simulink model "Neurofeedback_Fuzzy_MISO_Full_3x3"  (R2022a)
settings: Solver=VariableStepAuto  StartTime=0.0  StopTime=2700  RelTol=1e-3
libraries: dspsrcs4 x12, simulink x5, fuzblock x1
(part 2 of 2)

== matlab function Neurofeedback_Fuzzy_MISO_Full_3x3/Synthetic Human Agent/Noise Models/Physiological Noise_ Vasomotion ==
  settings: updateMethod=DISCRETE
  data: FreqSD input; HemoNoises output; FreqMean input; ResolutionStep input; timestamps input
function HemoNoises  = Neurofeedback_PhysiologicalNoise(FreqSD, FreqMean, ResolutionStep, timestamps)
%% Version V1
% Authors - Mario De Los Santos, Felipe Orihuela-Espina, Javier
% Herrera-Vega, Javier Andreu-Pérez
% Date - July 18th, 2022
% Email - madlsh3517@gmail.com
% Based on: Elwell et. al., 1999. Oscillations in cerebal haemodynamics.
%
%% Input Parameters
% FreqSD - Frequency standard deviation of the physiological noise. Scalar
% FreqMean - Frequency Mean of the physiological noise. Scalar
% Resolution Step - Sampling rate. Scalar
% Timestamps - Time sequence for the stimulus train. <1 x simulationLength>
% NRegions - Number of regions activated. Scalar.
%% Output Parameters
% 
% HemoNoises -  Noise generation for the hemodynamics signals.
%               <NRegions x simulationLength>
%
%% 

%Variables to ADD the noises to the models. 
% These variables divide the hemodynamics 
% inputs depending on the number of regions.
HemoNoises = 0;

%Calculation of the operative ranges to use
Initial =  FreqMean - 2 * FreqSD;
Ending = FreqMean + 2 * FreqSD + ResolutionStep;
Calsize =  (Ending - Initial)/ResolutionStep;
FrequencySet = linspace(Initial, Ending, Calsize);

amplitudeScaling = 1;
for i = 1:Calsize
    s = rng; %Rebot random seeed 
    %Random Amplitude
    %Centralized gaussian in the dispersion mean 
    %A = 0;
    A = amplitudeScaling * normrnd(FreqMean,FreqSD);
    %A = amplitudeScaling * randn(1);
  
    %Random phase
    theta = (2 * pi * normrnd(FreqMean, FreqSD) - pi );
  
    %Fundamental signal
    tmpSin = A * sin(pi * FrequencySet(1,i) * timestamps + theta);
    HemoNoises = HemoNoises + tmpSin;
end
%This section should be generalized but do the work for now.

== matlab function Neurofeedback_Fuzzy_MISO_Full_3x3/Synthetic Human Agent/Noise Models/Physiological Noise_Heart ==
  settings: updateMethod=DISCRETE
  data: FreqSD input; HemoNoises output; FreqMean input; ResolutionStep input; timestamps input
function HemoNoises  = Neurofeedback_PhysiologicalNoise(FreqSD, FreqMean, ResolutionStep, timestamps)
%% Version V1
% Authors - Mario De Los Santos, Felipe Orihuela-Espina, Javier
% Herrera-Vega, Javier Andreu-Pérez
% Date - July 18th, 2022
% Email - madlsh3517@gmail.com
% Based on: Elwell et. al., 1999. Oscillations in cerebal haemodynamics.
%
%% Input Parameters
% FreqSD - Frequency standard deviation of the physiological noise. Scalar
% FreqMean - Frequency Mean of the physiological noise. Scalar
% Resolution Step - Sampling rate. Scalar
% Timestamps - Time sequence for the stimulus train. <1 x simulationLength>
% NRegions - Number of regions activated. Scalar.
%% Output Parameters
% 
% HemoNoises -  Noise generation for the hemodynamics signals.
%               <NRegions x simulationLength>
%
%% 

%Variables to ADD the noises to the models. 
% These variables divide the hemodynamics 
% inputs depending on the number of regions.
HemoNoises = 0;
%
%Calculation of the operative ranges to use
Initial =  FreqMean - 2*FreqSD;
Ending = FreqMean +  2*FreqSD;
Calsize = (Ending - Initial - ResolutionStep)/ResolutionStep;
%Calsize = ResolutionStep;
FrequencySet = linspace(Initial, Ending, Calsize);

amplitudeScaling = 1;
theta = 0;
for i = 1:Calsize
    s = rng; %Rebot random seeed 
    %Random Amplitude
    %Centralized gaussian in the dispersion mean 
    %A = 0;
    A = amplitudeScaling * normrnd(FreqMean,FreqSD);
    %A = amplitudeScaling * rand(1);
    %Random phase
    %theta = 2 * pi * normrnd(FreqMean, FreqSD) - pi;
    
    %Fundamental signal
    tmpSin = A * sin(2*pi*(FrequencySet(1,i) * timestamps + theta));
    HemoNoises = HemoNoises + tmpSin;
end
%This section should be generalized but do the work for now.

== matlab function Neurofeedback_Fuzzy_MISO_Full_3x3/Error Function2/Error Function/ErrorFunction_GRG ==
  data: Bref input; E output size=1; Bobs input; Pref input; Pobs input; SHD input; w1_l input; errP output; errA output
function [E, errP, errA]  = ErrorFunction(Bref, Bobs, Pref, Pobs, SHD, w1_l)
    w1 = w1_l; %Use whatever values you like most. Threshold 

    w2 = 1 - w1;

    assert(all(size(Bref) == size(Bobs)));

    assert(size(Bref,1) == size(Bref,2));

    nChannels = size(Bref,1);

    BfullyConnected = ones(nChannels);

    BfullyDisconnected = zeros(nChannels);

   
    maxDiffSHD= sum(sum(xor(BfullyConnected,BfullyDisconnected))); %SHD
    errA = SHD/maxDiffSHD; %Normalize error in the connectivity
    %errP = (abs(Pref-Pobs))/abs(Pref);
    %tmp = Pref;
    errP = abs(Pref-Pobs)/max(abs(Pref),1);

    
E = (w1 * errA + w2 * errP);

== matlab function Neurofeedback_Fuzzy_MISO_Full_3x3/Synthetic Human Agent1/Hemodynamics/Rate Blood Volume/Fv_s ==
  data: Vj input; Vj_expphi output
function Vj_expphi = fcn(Vj)
phi = 0.32;
Vj_expphi = Vj.^(1/phi);

== matlab function Neurofeedback_Fuzzy_MISO_Full_3x3/Synthetic Human Agent1/Hemodynamics/Rate Blood Volume/Vj//Tjv ==
  data: Vj input; Vj_Tjv output
function Vj_Tjv = fcn(Vj)
    Tjv = 2*exp([0;1;0]);
    Tj = 2*exp([0;0.05;0.05]);
Vj_Tjv =(Tj.*Tjv.*Vj);

== matlab function Neurofeedback_Fuzzy_MISO_Full_3x3/Subsystem/getConnectivity_Validation1 ==
  data: D input; Bobs output; DQ output; Threshold input
function [Bobs,DQ]  = getConnectivity(D, Threshold)

    DQ = zeros(1, 3);
    DQ(1,1)=D(1,1);
    DQ(1,2)=D(1,2);
    DQ(1,3)=D(1,3);

    rThresh= Threshold; % [0..1] A threshold on the correlation.

    [~,nChannels, nHb]=size(DQ);

    C = nan(nChannels, nChannels, nHb); %Matrix of channel pairwise correlations;

    %This part of the algorithm is HIGHLY inefficient but it does the job for now
    %but might not be sufficiently fast for "real time" neurofeedback

    for iHb = 1:nHb
        for iCh=1:nChannels
            for jCh=iCh:nChannels

                if iCh == jCh

                 C(iCh,jCh,iHb) = 1;

                else

                 C(iCh,jCh,iHb) = xcorr2(DQ(:,iCh,iHb),DQ(:,jCh,iHb));

                end
            end

        end

    end

    %Threshold/Binarize C


    tmp = C > rThresh;

    %Finally "merge" accross Hb species

    Bobs = all(tmp,3); %Apply the AND function across Hb species.

== matlab function Neurofeedback_Fuzzy_MISO_Full_3x3/fNIRS Processing/Channel Organizer ==
  data: u input; y output
function y = fcn(u)

y = [1; 2; 3; 4; 5; 6];

y(1) = u(1,1);
y(2) = u(2,1);

y(3) = u(1,2);
y(4) = u(2,2);

y(5) = u(3,1);
y(6) = u(3,2);

== matlab function Neurofeedback_Fuzzy_MISO_Full_3x3/Connectivity_Regions3 ==
  data: Bobs input; B_00 output; B_01 output; B_02 output; B_10 output; B_11 output; B_12 output; B_20 output; B_21 output; B_22 output
function [B_00, B_01, B_02, B_10, B_11, B_12,  B_20, B_21, B_22] = fcn(Bobs)


B_00 = (Bobs(1,1));
B_01 = (Bobs(1,2));
B_02 = (Bobs(1,3));

B_10 = (Bobs(2,1));
B_11 = (Bobs(2,2));
B_12 = (Bobs(2,3));

B_20 = (Bobs(3,1));
B_21 = (Bobs(3,2));
B_22 = (Bobs(3,3));

== matlab function Neurofeedback_Fuzzy_MISO_Full_3x3/Subsystem/Incremental_Avg_Boot1/Reboot/MATLAB Function1 ==
  data: Timer input; Reset output; Cycle_time input; periods input
function Reset  = fcn(Timer, Cycle_time, periods)

temp = 0;
PCycles = zeros(periods,1);
for i = 1:periods
    PCycles(i) = i * Cycle_time;
    if (Timer >= PCycles(i) && Timer <= PCycles(i)+1)
        temp = 1;
        break
    else
        temp = 0;
    end
end 
Reset = temp;

== matlab function Neurofeedback_Fuzzy_MISO_Full_3x3/Subsystem/Incremental_Avg_Boot1/Reboot/MATLAB Function2 ==
  data: reset input; y_s input; y output
function y = fcn(reset, y_s)

if reset == 1
    y = 0;
else 
    y = (y_s + 1);
end

== matlab function Neurofeedback_Fuzzy_MISO_Full_3x3/Synthetic Human Agent1/Human_Pressure/Pressure Generator ==
  data: Zt input; Pobs output; t input
function Pobs = fcn(Zt, t)
    R=10000; %Resistor [Ohms];
    C= 2; %Capacitor [Faradays];
    V= Zt(2); %Voltage or system reference;
    Vc = V * (exp(-t/(R*C))); % Voltage at the capacitor  
    
Pobs = Vc;

== matlab function Neurofeedback_Fuzzy_MISO_Full_3x3/Synthetic Human Agent/Hemodynamics/Rate Blood Volume/Fv_s ==
  data: Vj input; Vj_expphi output
function Vj_expphi = fcn(Vj)
phi = 0.32;
Vj_expphi = Vj.^(1/phi);

== matlab function Neurofeedback_Fuzzy_MISO_Full_3x3/Synthetic Human Agent1/Human_Pressure/SENSOR ==
  data: Vout input; Pobs output
function Pobs  = PressureGenerator_sensor(Vout)

    Vcc = 50; %Considering 5V as a real sensor, the value is on mV
    Rf = 100; %Fixed resistor 10k ohms
    kgf = 0.1019716213; % 1N = 0.1019716213 kgf
    Fsr = 0;
    Fsrforce = 0;
    Fsr = (Vcc - Vout * Rf) / Vout;
    FsConductance = 1000000; %Sensor conductance in uOhms
    FsConductance = FsConductance / Fsr;
    if FsConductance <= 1000
        Fsrforce = FsConductance / 80; %Force on Newtons
    else
        Fsrforce = FsConductance - 1000;
        Fsrforce = Fsrforce / 30;
    end
    
Pobs = Fsrforce * kgf;

end

== matlab function Neurofeedback_Fuzzy_MISO_Full_3x3/Synthetic Human Agent1/Neurodynamics_Static/B_Dynamic1/MATLAB Function ==
  settings: updateMethod=DISCRETE
  data: B input; B_d output; U input; Th output; T input; Th_O input
function [B_d, Th]= fcn(B, U, T, Th_O)
B_d = zeros(3,3);
Th = [1 1 1 1; 1 1 1 1];
down = -1.1;
up = 1.1;
%Plasticity threshold
if T >= 0 && T <= 1
    x = rand(1, 4);
    x = sort(x);
    s = std(x);
    Th(1,:) = x;
    Th(2,:) = x + s;
else
    Th = Th_O;
end
db = B;
if U > Th(1,2) && U < Th(2, 2)
   dB = (up-down).*rand(3,3) + down;
   if(det(dB) > 0.25 && det(db) < 0.7)
       B_d = dB;
   else
       dB = (up-down).*rand(3,3) + down;
       B_d = dB;
   end
elseif U > Th(2,2) && U < Th(1,3)
   dB = (up-down).*rand(3,3) + down;
   if(det(dB) > 0 && det(db) < 0.25)
       B_d = dB;
   else
       dB = (up-down).*rand(3,3) + down;
       B_d = dB;
   end
else
    B_d = B;
end

== matlab function Neurofeedback_Fuzzy_MISO_Full_3x3/Synthetic Human Agent1/Neurodynamics_Static/Jt ==
  data: Zt input; U input; Jt output; B_input input; A_input input
function Jt = fcn(Zt, U, B_input, A_input)
   A = A_input;
   nRegions  = size(A,1);
   M = size(U,1); %nStimuli
   simulationLength = size(U,2);
   %NOTE: Consider that in case of have more than one stimulus, you must
   %change this. 
   B = B_input;
   T = zeros(nRegions); %nRegions x nRegions
    for t = 1:simulationLength
           for uu = 1:M % Sum (Uj * Bj)
               tmp = U(uu,t)*B(:,:,uu);
               T = -0.5*exp(T + tmp);  
           end
    end
    SI = diag(A);
    A =  A - diag(exp(SI) + SI);
Jt = (A*Zt) + (T*Zt);

== matlab function Neurofeedback_Fuzzy_MISO_Full_3x3/Synthetic Human Agent1/Noise Models/Gains calculator ==
  settings: updateMethod=DISCRETE
  data: PercentError input; Signal1_avgAmplitud input; Signal2_avgAmplitud input; Signal3_avgAmplitud input; Signal4_avgAmplitud input; Gain1 output; MaxAmplitudeHemodynamics input; Gain2 output; Gain3 output; Gain4 output
function [Gain1, Gain2, Gain3, Gain4]    = Noise_gains(PercentError, Signal1_avgAmplitud,Signal2_avgAmplitud ,Signal3_avgAmplitud,Signal4_avgAmplitud, MaxAmplitudeHemodynamics)

Gain1 = ((MaxAmplitudeHemodynamics / 100) * PercentError)/ Signal1_avgAmplitud;

Gain2 = ((MaxAmplitudeHemodynamics / 100) * PercentError)/ Signal2_avgAmplitud;

Gain3 = ((MaxAmplitudeHemodynamics / 100) * PercentError)/ Signal3_avgAmplitud;

Gain4 = ((MaxAmplitudeHemodynamics / 100) * PercentError)/ Signal4_avgAmplitud;

== matlab function Neurofeedback_Fuzzy_MISO_Full_3x3/Synthetic Human Agent1/Noise Models/Physiological Noise_ Breathing ==
  settings: updateMethod=DISCRETE
  data: FreqSD input; HemoNoises output; FreqMean input; ResolutionStep input; timestamps input
function HemoNoises  = Neurofeedback_PhysiologicalNoise(FreqSD, FreqMean, ResolutionStep, timestamps)
%% Version V1
% Authors - Mario De Los Santos, Felipe Orihuela-Espina, Javier
% Herrera-Vega, Javier Andreu-Pérez
% Date - July 18th, 2022
% Email - madlsh3517@gmail.com
% Based on: Elwell et. al., 1999. Oscillations in cerebal haemodynamics.
%
%% Input Parameters
% FreqSD - Frequency standard deviation of the physiological noise. Scalar
% FreqMean - Frequency Mean of the physiological noise. Scalar
% Resolution Step - Sampling rate. Scalar
% Timestamps - Time sequence for the stimulus train. <1 x simulationLength>
% NRegions - Number of regions activated. Scalar.
%% Output Parameters
% 
% HemoNoises -  Noise generation for the hemodynamics signals.
%               <NRegions x simulationLength>
%
%% 

%Variables to ADD the noises to the models. 
% These variables divide the hemodynamics 
% inputs depending on the number of regions.
HemoNoises = 0;

%Calculation of the operative ranges to use
Initial =  FreqMean - 2 * FreqSD;
Ending = FreqMean + 2 * FreqSD;
Calsize =  (Ending - Initial - ResolutionStep)/ResolutionStep;
FrequencySet = linspace(Initial, Ending, Calsize);

amplitudeScaling = 1;
for i = 1:Calsize
    s = rng; %Rebot random seeed 
    %Random Amplitude
    %Centralized gaussian in the dispersion mean 
    %A = 0;
    L = normrnd(FreqMean, FreqSD);
    A = amplitudeScaling * L;
  
    %Random phase
    theta = (2 * pi * L - pi );
  
    %Fundamental signal
    tmpSin = A * sin(pi * FrequencySet(1,i) * timestamps + theta);
    HemoNoises = HemoNoises + tmpSin;
end
%This section should be generalized but do the work for now.

== matlab function Neurofeedback_Fuzzy_MISO_Full_3x3/Synthetic Human Agent1/Noise Models/Physiological Noise_ Breathing1 ==
  settings: updateMethod=DISCRETE
  data: FreqSD input; HemoNoises output; FreqMean input; ResolutionStep input; timestamps input
function HemoNoises  = Neurofeedback_PhysiologicalNoise(FreqSD, FreqMean, ResolutionStep, timestamps)
%% Version V1
% Authors - Mario De Los Santos, Felipe Orihuela-Espina, Javier
% Herrera-Vega, Javier Andreu-Pérez
% Date - July 18th, 2022
% Email - madlsh3517@gmail.com
% Based on: Elwell et. al., 1999. Oscillations in cerebal haemodynamics.
%
%% Input Parameters
% FreqSD - Frequency standard deviation of the physiological noise. Scalar
% FreqMean - Frequency Mean of the physiological noise. Scalar
% Resolution Step - Sampling rate. Scalar
% Timestamps - Time sequence for the stimulus train. <1 x simulationLength>
% NRegions - Number of regions activated. Scalar.
%% Output Parameters
% 
% HemoNoises -  Noise generation for the hemodynamics signals.
%               <NRegions x simulationLength>
%
%% 

%Variables to ADD the noises to the models. 
% These variables divide the hemodynamics 
% inputs depending on the number of regions.
HemoNoises = 0;

%Calculation of the operative ranges to use
Initial =  FreqMean - 2 * FreqSD;
Ending = FreqMean + 2 * FreqSD;
Calsize =  (Ending - Initial)/ResolutionStep;
FrequencySet = linspace(Initial, Ending, Calsize);

amplitudeScaling = 1;
for i = 1:Calsize
    s = rng; %Rebot random seeed 
    %Random Amplitude
    %Centralized gaussian in the dispersion mean 
    %A = 0;
    L = normrnd(FreqMean, FreqSD);
    A = amplitudeScaling * L;
  
    %Random phase
    theta = 0;
  
    %Fundamental signal
    tmpSin = A * sin((pi * FrequencySet(1,i) * timestamps + theta)*2*pi);
    HemoNoises = HemoNoises + tmpSin;
end
%This section should be generalized but do the work for now.

== matlab function Neurofeedback_Fuzzy_MISO_Full_3x3/fNIRS Processing/MATLAB Function2 ==
  data: e_coefficients input; A output; DPF input; Distance input
function A  = A(e_coefficients, DPF, Distance)
%Molar extinction coefficients 
%Considering the wavelengths of the STak implentation, we need to use
% 780nm and 850nm

%780nm = [735.8251 1104.715];
%850nm = [1159.306 785.8993];
%e_coefficients = [735.8251 1104.715;
 %                   1159.306 785.8993];

% https://mail.nmr.mgh.harvard.edu/pipermail//homer-users/2006-July/000124.html
%Differential Path Lenght
%NOTE: need to confirm this, I'm taking the values from an old
%implementation
%DPF = [10.3; 8.4];

%Distance; this is an assumption of 3cm
%Distance = 3;
A = [e_coefficients(1, 1)*Distance*DPF(1), e_coefficients(1, 2)*Distance*DPF(1);...
    e_coefficients(2, 1)*Distance*DPF(2), e_coefficients(2, 1)*Distance*DPF(2)];

== matlab function Neurofeedback_Fuzzy_MISO_Full_3x3/Synthetic Human Agent1/Noise Models/Physiological Noise_ Vasomotion ==
  settings: updateMethod=DISCRETE
  data: FreqSD input; HemoNoises output; FreqMean input; ResolutionStep input; timestamps input
function HemoNoises  = Neurofeedback_PhysiologicalNoise(FreqSD, FreqMean, ResolutionStep, timestamps)
%% Version V1
% Authors - Mario De Los Santos, Felipe Orihuela-Espina, Javier
% Herrera-Vega, Javier Andreu-Pérez
% Date - July 18th, 2022
% Email - madlsh3517@gmail.com
% Based on: Elwell et. al., 1999. Oscillations in cerebal haemodynamics.
%
%% Input Parameters
% FreqSD - Frequency standard deviation of the physiological noise. Scalar
% FreqMean - Frequency Mean of the physiological noise. Scalar
% Resolution Step - Sampling rate. Scalar
% Timestamps - Time sequence for the stimulus train. <1 x simulationLength>
% NRegions - Number of regions activated. Scalar.
%% Output Parameters
% 
% HemoNoises -  Noise generation for the hemodynamics signals.
%               <NRegions x simulationLength>
%
%% 

%Variables to ADD the noises to the models. 
% These variables divide the hemodynamics 
% inputs depending on the number of regions.
HemoNoises = 0;

%Calculation of the operative ranges to use
Initial =  FreqMean - 2 * FreqSD;
Ending = FreqMean + 2 * FreqSD + ResolutionStep;
Calsize =  (Ending - Initial)/ResolutionStep;
FrequencySet = linspace(Initial, Ending, Calsize);

amplitudeScaling = 1;
for i = 1:Calsize
    s = rng; %Rebot random seeed 
    %Random Amplitude
    %Centralized gaussian in the dispersion mean 
    %A = 0;
    A = amplitudeScaling * normrnd(FreqMean,FreqSD);
    %A = amplitudeScaling * randn(1);
  
    %Random phase
    theta = (2 * pi * normrnd(FreqMean, FreqSD) - pi );
  
    %Fundamental signal
    tmpSin = A * sin(pi * FrequencySet(1,i) * timestamps + theta);
    HemoNoises = HemoNoises + tmpSin;
end
%This section should be generalized but do the work for now.

== matlab function Neurofeedback_Fuzzy_MISO_Full_3x3/Synthetic Human Agent1/Noise Models/Physiological Noise_Heart ==
  settings: updateMethod=DISCRETE
  data: FreqSD input; HemoNoises output; FreqMean input; ResolutionStep input; timestamps input
function HemoNoises  = Neurofeedback_PhysiologicalNoise(FreqSD, FreqMean, ResolutionStep, timestamps)
%% Version V1
% Authors - Mario De Los Santos, Felipe Orihuela-Espina, Javier
% Herrera-Vega, Javier Andreu-Pérez
% Date - July 18th, 2022
% Email - madlsh3517@gmail.com
% Based on: Elwell et. al., 1999. Oscillations in cerebal haemodynamics.
%
%% Input Parameters
% FreqSD - Frequency standard deviation of the physiological noise. Scalar
% FreqMean - Frequency Mean of the physiological noise. Scalar
% Resolution Step - Sampling rate. Scalar
% Timestamps - Time sequence for the stimulus train. <1 x simulationLength>
% NRegions - Number of regions activated. Scalar.
%% Output Parameters
% 
% HemoNoises -  Noise generation for the hemodynamics signals.
%               <NRegions x simulationLength>
%
%% 

%Variables to ADD the noises to the models. 
% These variables divide the hemodynamics 
% inputs depending on the number of regions.
HemoNoises = 0;
%
%Calculation of the operative ranges to use
Initial =  FreqMean - 2*FreqSD;
Ending = FreqMean +  2*FreqSD;
Calsize = (Ending - Initial - ResolutionStep)/ResolutionStep;
%Calsize = ResolutionStep;
FrequencySet = linspace(Initial, Ending, Calsize);

amplitudeScaling = 1;
theta = 0;
for i = 1:Calsize
    s = rng; %Rebot random seeed 
    %Random Amplitude
    %Centralized gaussian in the dispersion mean 
    %A = 0;
    A = amplitudeScaling * normrnd(FreqMean,FreqSD);
    %A = amplitudeScaling * rand(1);
    %Random phase
    %theta = 2 * pi * normrnd(FreqMean, FreqSD) - pi;
    
    %Fundamental signal
    tmpSin = A * sin(2*pi*(FrequencySet(1,i) * timestamps + theta));
    HemoNoises = HemoNoises + tmpSin;
end
%This section should be generalized but do the work for now.

== matlab function Neurofeedback_Fuzzy_MISO_Full_3x3/Synthetic Human Agent1/Optics_1 ==
  data: DH input; DQ input; Y output; tempDHQ output
function [Y, tempDHQ]   = Optical_Changes(DH, DQ)
%% Version V1
% Authors - Mario De Los Santos, Felipe Orihuela-Espina, Javier Herrara-Vega
% Date - March, 2022
% Email - madlsh3517@gmail.com
% Based on: 2015 Stak DCM for fNIRS.
%
%% Input Parameters
% DQ - HbR - Rate of deoxy-hemoglobin
% DH - HbT - Total Hemoglobin
%
%% Output Parameters
% y- optical density changes 
%
%% 

%Using simulink is not possible to have a dynamic matrix that we can
%iterate based on the nRegions variable, but you could easly replace the
%number of regions in the variable "Regions" according your needs
Regions = 3;
Y = zeros(2, Regions);
tempDHQ = zeros(2, Regions);
% We are using as L1 = 780nm and as L2 = 850nm (same as STak for the
% second one)
%Based on: Giannoni, L., Lange, F., & Tachtsidis, I. (2020). Investigation of the quantification 
% of hemoglobin and cytochrome-c-oxidase in the exposed cortex with near-infrared hyperspectral imaging: 
% a simulation study. Journal of biomedical optics, 25(4), 046001.


F_P =[(0.0007358251*7.5) (0.001104715*6.5);
      (0.001159306*7.5) (0.0007858993*6.5)];
%F_P = [(735.8251*7.5), (1104.715*7.5); (1159.306*7.5), (785.8993*7.5)];
%Itereation between regions, nRegions is given as constant by the user.

    tempDHQ(1,1) = DH(1);
    tempDHQ(1,2) = DH(2);
    tempDHQ(1,3) = DH(3);

    tempDHQ(2,1) = DQ(1);
    tempDHQ(2,2) = DQ(2);
    tempDHQ(2,3) = DQ(3);


    Y(:,1) = F_P * tempDHQ(:,1);
    Y(:,2) = F_P * tempDHQ(:,2);
    Y(:,3) = F_P * tempDHQ(:,3);

== matlab function Neurofeedback_Fuzzy_MISO_Full_3x3/Synthetic Human Agent1/Visual Interpretation ==
  data: Visual_Stimulus input; Response output; t input
function Response = fcn(Visual_Stimulus, t)
    R=17.5; %Resistor [Ohms] 10k 
    C= 0.65; %Capacitor [Faradays] 1mF
    V= Visual_Stimulus; %Voltage or system reference;
    Vc = V * (1- exp(-t/(R*C))); % Voltage at the capacitor  
    
Response = Vc;

== matlab function Neurofeedback_Fuzzy_MISO_Full_3x3/Synthetic Human Agent/Hemodynamics/Rate Blood Volume/Vj//Tjv ==
  data: Vj input; Vj_Tjv output
function Vj_Tjv = fcn(Vj)
    Tjv = 2*exp([0;1]);
    Tj = 2*exp([0;0.05]);
Vj_Tjv =(Tj.*Tjv.*Vj);

== matlab function Neurofeedback_Fuzzy_MISO_Full_3x3/Synthetic Human Agent/Human_Pressure/Pressure Generator ==
  data: Zt input; Pobs output; t input
function Pobs = fcn(Zt, t)
    R=10000; %Resistor [Ohms];
    C= 2; %Capacitor [Faradays];
    V= Zt(1); %Voltage or system reference;
    Vc = V * (exp(-t/(R*C))); % Voltage at the capacitor  
    
Pobs = Vc;

== matlab function Neurofeedback_Fuzzy_MISO_Full_3x3/Synthetic Human Agent/Human_Pressure/SENSOR ==
  data: Vout input; Pobs output
function Pobs  = PressureGenerator_sensor(Vout)

    Vcc = 50; %Considering 5V as a real sensor, the value is on mV
    Rf = 100; %Fixed resistor 10k ohms
    kgf = 0.1019716213; % 1N = 0.1019716213 kgf
    Fsr = 0;
    Fsrforce = 0;
    Fsr = (Vcc - Vout * Rf) / Vout;
    FsConductance = 1000000; %Sensor conductance in uOhms
    FsConductance = FsConductance / Fsr;
    if FsConductance <= 1000
        Fsrforce = FsConductance / 80; %Force on Newtons
    else
        Fsrforce = FsConductance - 1000;
        Fsrforce = Fsrforce / 30;
    end
    
Pobs = Fsrforce * kgf;

end

== matlab function Neurofeedback_Fuzzy_MISO_Full_3x3/Synthetic Human Agent/Neurodynamics_Static/Jt ==
  data: Zt input; U input; Jt output; B_input input; A_input input
function Jt = fcn(Zt, U, B_input, A_input)
   A = A_input;
   nRegions  = size(A,1);
   M = size(U,1); %nStimuli
   simulationLength = size(U,2);
   %NOTE: Consider that in case of have more than one stimulus, you must
   %change this. 
   B = B_input;
   T = zeros(nRegions); %nRegions x nRegions
    for t = 1:simulationLength
           for uu = 1:M % Sum (Uj * Bj)
               tmp = U(uu,t)*B(:,:,uu);
               T = -0.5*exp(T + tmp);  
           end
    end
    SI = diag(A);
    A =  A - diag(exp(SI) + SI);
Jt = (A*Zt) + (T*Zt);

== matlab function Neurofeedback_Fuzzy_MISO_Full_3x3/Synthetic Human Agent/Optics_ ==
  data: nRegions input; DH input; DQ input; Y output; tempDHQ output
function [Y, tempDHQ]   = Optical_Changes(nRegions,DH, DQ)
%% Version V1
% Authors - Mario De Los Santos, Felipe Orihuela-Espina, Javier Herrara-Vega
% Date - March, 2022
% Email - madlsh3517@gmail.com
% Based on: 2015 Stak DCM for fNIRS.
%
%% Input Parameters
% DQ - HbR - Rate of deoxy-hemoglobin
% DH - HbT - Total Hemoglobin
%
%% Output Parameters
% y- optical density changes 
%
%% 

%Using simulink is not possible to have a dynamic matrix that we can
%iterate based on the nRegions variable, but you could easly replace the
%number of regions in the variable "Regions" according your needs
Regions = 2;
Y = zeros(Regions,Regions);
Ytemp1 = zeros(Regions,1);
Ytemp2 = zeros(Regions,1);
tempDHQ = zeros(Regions, 2);

%Debug temporal
L1 = zeros(Regions, 1);
L2 = zeros(Regions, 1);

% We are using as L1 = 780nm and as L2 = 850nm (same as STak for the
% second one)
%Based on: Giannoni, L., Lange, F., & Tachtsidis, I. (2020). Investigation of the quantification 
% of hemoglobin and cytochrome-c-oxidase in the exposed cortex with near-infrared hyperspectral imaging: 
% a simulation study. Journal of biomedical optics, 25(4), 046001.


F_P =[(0.0007358251*7.5) (0.001104715*6.5);
      (0.001159306*7.5) (0.0007858993*6.5)];
%F_P = [(735.8251*7.5), (1104.715*7.5); (1159.306*7.5), (785.8993*7.5)];
%Itereation between regions, nRegions is given as constant by the user.

    tempDHQ(1,1) = DH(1);
    tempDHQ(1,2) = DH(2);

    tempDHQ(2,1) = DQ(1);
    tempDHQ(2,2) = DQ(2);


    Ytemp1 = F_P * tempDHQ(:,1);
    Ytemp2 = F_P * tempDHQ(:,2);

    Y(:,1) = Ytemp1;
    Y(:,2) = Ytemp2;

% L1(1,1) = Y(1,1);
% L1(2,1) = Y(1,2);
% 
% L2(1,1) = Y(2,1);
% L2(2,1) = Y(2,2);

== matlab function Neurofeedback_Fuzzy_MISO_Full_3x3/Error Function2/Error Function/MATLAB Function(err2)_Saturated ==
  data: Bref input; E output size=1; Bobs input; Pref input; Pobs input; SHD input; w1_l input; errP output; errA output
function [E, errP, errA]  = ErrorFunction(Bref, Bobs, Pref, Pobs, SHD, w1_l)
    w1 = w1_l; %Use whatever values you like most. Threshold 

    w2 = 1 - w1;

    assert(all(size(Bref) == size(Bobs)));

    assert(size(Bref,1) == size(Bref,2));

    nChannels = size(Bref,1);

    BfullyConnected = ones(nChannels);

    BfullyDisconnected = zeros(nChannels);

   
    maxDiffSHD= sum(sum(xor(BfullyConnected,BfullyDisconnected))); %SHD
    errA = SHD/maxDiffSHD; %Normalize error in the connectivity
    %errP = (abs(Pref-Pobs))/abs(Pref);
    %tmp = Pref;
    errP = 0;
    if Pref == 0
        Pref = 0.0005;
    else
        %errP = abs(Pref-Pobs)/abs(Pref);
        errP = exp (1 / abs(Pref-Pobs)/abs(Pref));
      if errP > 1
            errP = 1;
      end
    end
    %errP = (abs(Pref-Pobs))/abs(tmp);
    
    
E = (w1 * errA + w2 * errP);

== matlab function Neurofeedback_Fuzzy_MISO_Full_3x3/Synthetic Human Agent/Neurodynamics_Static/B_Dynamic/MATLAB Function ==
  settings: updateMethod=DISCRETE
  data: B input; B_d output; U input; Th output; T input; Th_O input
function [B_d, Th]= fcn(B, U, T, Th_O)
B_d = [0 0; 0 0];
Th = [1 1 1 1; 1 1 1 1];
down = -1;
up = 1;
%Plasticity threshold
if T >= 0 && T <= 1
    x = rand(1, 4);
    x = sort(x);
    s = std(x);
    Th(1,:) = x;
    Th(2,:) = x + s;
else
    Th = Th_O;
end
db = B;
if U > Th(1,2) && U < Th(2, 2)
   dB = (up-down).*rand(3,3) + down;
   if(det(dB) > 0.3 && det(db) < 0.5)
       B_d = dB;
   else
       dB = (up-down).*rand(3,3) + down;
       B_d = dB;
   end
elseif U > Th(2,2) && U < Th(1,3)
   dB = (up-down).*rand(3,3) + down;
   if(det(dB) > 0 && det(db) < 0.3)
       B_d = dB;
   else
       dB = (up-down).*rand(3,3) + down;
       B_d = dB;
   end
else
    B_d = B;
end

== matlab function Neurofeedback_Fuzzy_MISO_Full_3x3/Synthetic Human Agent/DH and DQ/MATLAB Function1 ==
  data: DH1 input; H output; DH2 input; DQ1 input; DQ2 input
function H = hemo(DH1, DH2, DQ1, DQ2)
H = zeros(1,4);

H(1,1) = DQ1;
H(1,2) = DQ2;
H(1,3) = DH1;
H(1,4) = DH2;

== matlab function Neurofeedback_Fuzzy_MISO_Full_3x3/Error Function2/Error Function/Error_SHD ==
  data: Aref input; val output; Aobs input; matrix output
function [val,matrix]=SHD(Aref,Aobs)

val = sum(sum(xor(Aref,Aobs)));
matrix = xor(Aref,Aobs);

== matlab function Neurofeedback_Fuzzy_MISO_Full_3x3/Synthetic Human Agent/Hemodynamics/Efp ==
  data: fjin input; Efp output
function Efp= fcn(fjin)

Efp = (1 - (1 - 0.32).^ (1 ./ fjin))/0.32;

== matlab function Neurofeedback_Fuzzy_MISO_Full_3x3/fNIRS Processing/Modified Beer Lamber Law ==
  data: OD input; Hemodynamics output; A input
function Hemodynamics = MBLL(OD, A)

% B = zeros(2,2);
% 
% B(1, 1) = Delta1(1, 1);
% B(1, 2) = Delta1(2, 1);
% 
% B(2, 1) = Delta2(1, 1);
% B(2, 2) = Delta2(2, 1);

Hemodynamics = (A\OD)';
